simulink model "ctrl_custom_4corner_automatic"  (R2016b)
settings: Solver=ode4  StartTime=0.0  StopTime=inf  FixedStep=0.01  RelTol=1e-3  EnableMultiTasking=on
values from neighbouring files (symbols this model uses):
  alpha = R_T*Eta_t_dot - K1*z_1    [Immersion.m]
undefined symbols (not defined in the file or in its folder): T_pinv_m
libraries: marine_gnc x6, simulink x1
(part 5 of 5)

== system ctrl_custom_4corner_automatic/Complete MPAC1/MPAC Vel/zeta_phi ==
  Constant : Constant  Value=1.2
  Mux : Mux  Inputs=3
  zeta_phi_1 : S-Function  Priority=2  FunctionName=NIVeriStandIO  Parameters=width dtype portnum stime stype btype  SFunctionDeploymentMode=off  EnableBusSupport=off  mask(NI VeriStand Inport){portnum=2, width=-1, stime=-1, dtype=auto, stype=auto, btype=1}
      mask prompts: portnum "Port number:"; width "Port dimensions (-1 for dynamically sized):"; stime "Sample time (-1 for inherited):"; dtype "Data type:"; stype "Signal type:"; btype "Block type:"
      mask help: Use this inport on any level of nested subsystems to allow NI VeriStand software to map signals to it.
      mask init:
      | NIVeriStandIO_init;
      settings: CopyFcn=NIVeriStand_MDL_functions('', 'IO_copy');  DeleteFcn=NIVeriStand_MDL_functions('', 'IO_delete');  MoveFcn=set_param(gcb, 'Mask', 'on');
      mask Callback portnum: NIVeriStand_MDL_functions('', 'IO_setportnum');
      mask TypeOptions dtype: auto | double | single | int8 | uint8 | int16 | uint16 | int32 | uint32 | boolean
      mask Callback dtype: NIVeriStand_MDL_functions('', 'IO_booleansignal');
      mask TypeOptions stype: auto | real | complex
      mask Display:
      | patch([-x x], [-y y], [.90980 .81960 .32156]);
      | plot([xrad -x x xrad], [yrad -y y yrad]);
      | fprintf('NI In%d', portnum);
  zeta_phi_2 : S-Function  Priority=3  FunctionName=NIVeriStandIO  Parameters=width dtype portnum stime stype btype  SFunctionDeploymentMode=off  EnableBusSupport=off  mask(NI VeriStand Inport){portnum=3, width=-1, stime=-1, dtype=auto, stype=auto, btype=1}
      mask prompts: portnum "Port number:"; width "Port dimensions (-1 for dynamically sized):"; stime "Sample time (-1 for inherited):"; dtype "Data type:"; stype "Signal type:"; btype "Block type:"
      mask help: Use this inport on any level of nested subsystems to allow NI VeriStand software to map signals to it.
      mask init:
      | NIVeriStandIO_init;
      settings: CopyFcn=NIVeriStand_MDL_functions('', 'IO_copy');  DeleteFcn=NIVeriStand_MDL_functions('', 'IO_delete');  MoveFcn=set_param(gcb, 'Mask', 'on');
      mask Callback portnum: NIVeriStand_MDL_functions('', 'IO_setportnum');
      mask TypeOptions dtype: auto | double | single | int8 | uint8 | int16 | uint16 | int32 | uint32 | boolean
      mask Callback dtype: NIVeriStand_MDL_functions('', 'IO_booleansignal');
      mask TypeOptions stype: auto | real | complex
      mask Display:
      | patch([-x x], [-y y], [.90980 .81960 .32156]);
      | plot([xrad -x x xrad], [yrad -y y yrad]);
      | fprintf('NI In%d', portnum);
  zeta_phi_3 : S-Function  Priority=1  FunctionName=NIVeriStandIO  Parameters=width dtype portnum stime stype btype  SFunctionDeploymentMode=off  EnableBusSupport=off  mask(NI VeriStand Inport){portnum=1, width=-1, stime=-1, dtype=auto, stype=auto, btype=1}
      mask prompts: portnum "Port number:"; width "Port dimensions (-1 for dynamically sized):"; stime "Sample time (-1 for inherited):"; dtype "Data type:"; stype "Signal type:"; btype "Block type:"
      mask help: Use this inport on any level of nested subsystems to allow NI VeriStand software to map signals to it.
      mask init:
      | NIVeriStandIO_init;
      settings: CopyFcn=NIVeriStand_MDL_functions('', 'IO_copy');  DeleteFcn=NIVeriStand_MDL_functions('', 'IO_delete');  MoveFcn=set_param(gcb, 'Mask', 'on');
      mask Callback portnum: NIVeriStand_MDL_functions('', 'IO_setportnum');
      mask TypeOptions dtype: auto | double | single | int8 | uint8 | int16 | uint16 | int32 | uint32 | boolean
      mask Callback dtype: NIVeriStand_MDL_functions('', 'IO_booleansignal');
      mask TypeOptions stype: auto | real | complex
      mask Display:
      | patch([-x x], [-y y], [.90980 .81960 .32156]);
      | plot([xrad -x x xrad], [yrad -y y yrad]);
      | fprintf('NI In%d', portnum);
  zeta_phi : Outport
  wires:
  zeta_phi_1/1 -> Mux/1
  zeta_phi_3/1 -> Mux/3
  zeta_phi_2/1 -> Mux/2
  Constant/1 -> zeta_phi/1

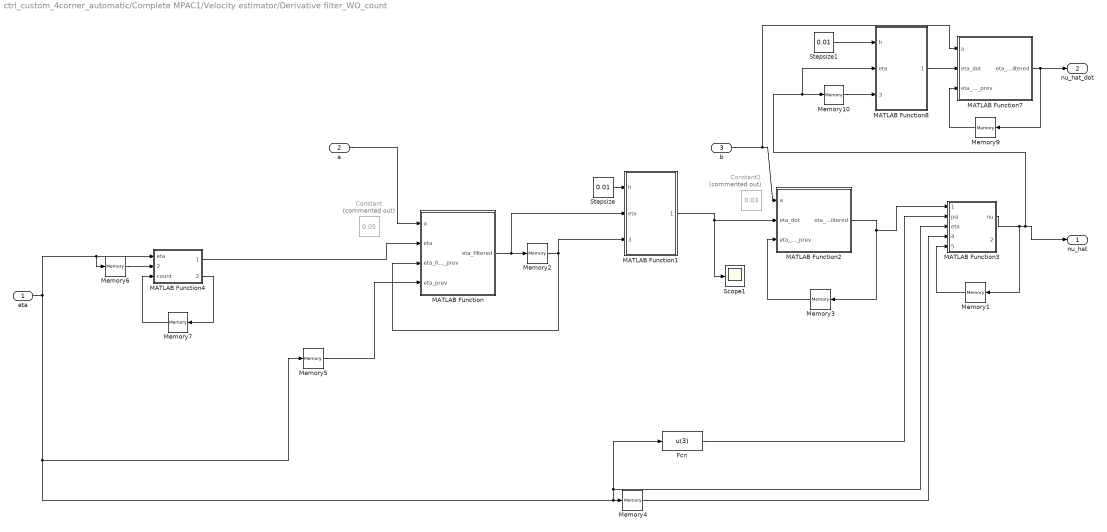
== system ctrl_custom_4corner_automatic/Complete MPAC1/Velocity estimator/Derivative filter_WO_count ==
  eta : Inport
  a : Inport  Port=2
  b : Inport  Port=3
  Constant : Constant  Commented=on  Value=0.05
  Constant2 : Constant  Commented=on  Value=0.03
  Fcn : Fcn  Expr=u(3)
  MATLAB Function : MATLAB Function  TreatAsAtomicUnit=on
  MATLAB Function1 : MATLAB Function  TreatAsAtomicUnit=on
  MATLAB Function2 : MATLAB Function  TreatAsAtomicUnit=on
  MATLAB Function3 : MATLAB Function  TreatAsAtomicUnit=on
  MATLAB Function4 : MATLAB Function  TreatAsAtomicUnit=on
  MATLAB Function7 : MATLAB Function  TreatAsAtomicUnit=on
  MATLAB Function8 : MATLAB Function  TreatAsAtomicUnit=on
  Memory{1..6,9..10} (8 alike) : Memory  X0=[0 0 0]
  Memory7 : Memory
  Scope1 : Scope
  Stepsize : Constant  Value=0.01
  Stepsize1 : Constant  Value=0.01
  nu_hat : Outport
  nu_hat_dot : Outport  Port=2
  wires:
  MATLAB Function7/1(eta_dot_filtered) -> Memory9/1, nu_hat_dot/1
  MATLAB Function4/2(count_out) -> Memory7/1
  Memory7/1 -> MATLAB Function4/3(count)
  Memory6/1 -> MATLAB Function4/2(eta_prev)
  MATLAB Function4/1(eta_out) -> MATLAB Function/2(eta)
  Stepsize1/1 -> MATLAB Function8/1(h)
  Memory10/1 -> MATLAB Function8/3(eta_prev)
  MATLAB Function8/1(eta_dot) -> MATLAB Function7/2(eta_dot)
  Memory9/1 -> MATLAB Function7/3(eta_dot_filtered_prev)
  eta/1 -> MATLAB Function4/1(eta), Memory6/1, Memory4/1, MATLAB Function3/3(eta), Fcn/1, Memory5/1
  Memory5/1 -> MATLAB Function/4(eta_prev)
  MATLAB Function3/1(nu) -> nu_hat/1, Memory10/1, MATLAB Function8/2(eta), Memory1/1
  Memory4/1 -> MATLAB Function3/4(prev_eta)
  Memory1/1 -> MATLAB Function3/5(prev_nu)
  MATLAB Function/1(eta_filtered) -> Memory2/1, MATLAB Function1/2(eta)
  b/1 -> MATLAB Function2/1(a), MATLAB Function7/1(a)
  a/1 -> MATLAB Function/1(a)
  Memory3/1 -> MATLAB Function2/3(eta_dot_filtered_prev)
  MATLAB Function2/1(eta_dot_filtered) -> Memory3/1, MATLAB Function3/1(eta_dot)
  MATLAB Function1/1(eta_dot) -> MATLAB Function2/2(eta_dot), Scope1/1
  Memory2/1 -> MATLAB Function/3(eta_filtered_prev), MATLAB Function1/3(eta_prev)
  Stepsize/1 -> MATLAB Function1/1(h)
  Fcn/1 -> MATLAB Function3/2(psi)

== system ctrl_custom_4corner_automatic/Saturation/MRS_num/LP ==
  In1 : Inport
  Gain1 : Gain  Gain=2  Multiplication=Matrix(K*u)
  Integrator : Integrator  InitialCondition=[0;0;0]
  Sum2 : Sum  Inputs=|+-
  Out1 : Outport
  wires:
  Sum2/1 -> Gain1/1
  In1/1 -> Sum2/1
  Integrator/1 -> Sum2/2, Out1/1
  Gain1/1 -> Integrator/1

== system ctrl_custom_4corner_automatic/Saturation1/MRS_num/LP ==
  In1 : Inport
  Gain1 : Gain  Gain=2  Multiplication=Matrix(K*u)
  Integrator : Integrator  InitialCondition=[0;0;0]
  Sum2 : Sum  Inputs=|+-
  Out1 : Outport
  wires:
  Gain1/1 -> Integrator/1
  Integrator/1 -> Out1/1, Sum2/2
  In1/1 -> Sum2/1
  Sum2/1 -> Gain1/1

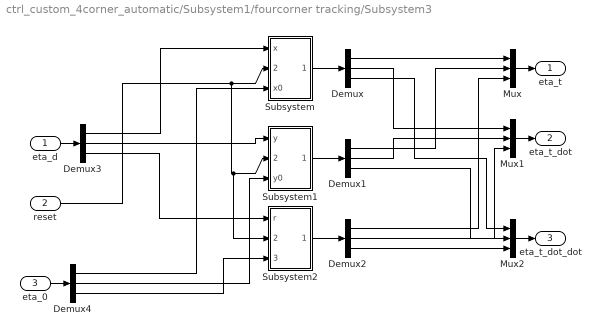
== system ctrl_custom_4corner_automatic/Subsystem1/fourcorner tracking/Subsystem3 ==
  eta_d : Inport
  reset : Inport  Port=2
  eta_0 : Inport  Port=3
  Demux{,1..4} (5 alike) : Demux  Outputs=3
  Mux : Mux  Inputs=3
  Mux1 : Mux  Inputs=3
  Mux2 : Mux  Inputs=3
  Subsystem : Subsystem
  Subsystem1 : Subsystem
  Subsystem2 : Subsystem
  eta_t : Outport  PortDimensions=3
  eta_t_dot : Outport  Port=2  PortDimensions=3
  eta_t_dot_dot : Outport  Port=3  PortDimensions=3
  wires:
  Subsystem1/1(y,yd,ydd) -> Demux1/1
  Subsystem2/1(y,yd,ydd) -> Demux2/1
  Subsystem/1(x,xd,xdd) -> Demux/1
  Demux/3 -> Mux2/1
  eta_d/1 -> Demux3/1
  Mux1/1 -> eta_t_dot/1
  Demux/1 -> Mux/1
  Mux2/1 -> eta_t_dot_dot/1
  Demux3/1 -> Subsystem/1(x)
  Demux1/3 -> Mux2/2
  Demux2/3 -> Mux2/3
  Demux1/1 -> Mux/2
  Demux3/2 -> Subsystem1/1(y)
  Demux3/3 -> Subsystem2/1(r)
  Demux2/2 -> Mux1/3
  Demux1/2 -> Mux1/2
  reset/1 -> Subsystem2/2(reset), Subsystem1/2(reset), Subsystem/2(reset)
  Mux/1 -> eta_t/1
  Demux/2 -> Mux1/1
  Demux2/1 -> Mux/3
  Demux4/3 -> Subsystem2/3(psi0)
  Demux4/2 -> Subsystem1/3(y0)
  Demux4/1 -> Subsystem/3(x0)
  eta_0/1 -> Demux4/1

== system ctrl_custom_4corner_automatic/Complete MPAC1/MPAC/Subsystem/10HZ ==
  In1 : Inport
  MATLAB Function : MATLAB Function  TreatAsAtomicUnit=on
  Memory : Memory
  Memory1 : Memory
  Out1 : Outport
  wires:
  Memory/1 -> MATLAB Function/3(i)
  MATLAB Function/2(i_out) -> Memory/1
  Memory1/1 -> MATLAB Function/2(nu_current)
  MATLAB Function/1(nu_10) -> Out1/1, Memory1/1
  In1/1 -> MATLAB Function/1(nu)

== system ctrl_custom_4corner_automatic/Subsystem1/fourcorner tracking/Subsystem3/Subsystem ==
  x : Inport
  reset : Inport  Port=2
  x0 : Inport  Port=3
  Constant : Constant  Value=0
  Gain1 : Gain  Gain=[0 0 0.0017]'  Multiplication=Matrix(K*u)
  Gain2 : Gain  Gain=[1 0 0;0 1 0;0 0 1]  Multiplication=Matrix(K*u)
  Gain3 : Gain  Gain=[0 1 0;0 0 1;-0.0017 -0.049 -0.408]  Multiplication=Matrix(K*u)
  Integrator : Integrator  ExternalReset=either  InitialConditionSource=external
  Mux : Mux  Inputs=3
  Sum : Sum  Inputs=|++
  x,xd,xdd : Outport  PortDimensions=3
  wires:
  Gain1/1 -> Sum/1
  x/1 -> Gain1/1
  Integrator/1 -> Gain2/1, Gain3/1
  Sum/1 -> Integrator/1
  Gain2/1 -> x,xd,xdd/1
  Mux/1 -> Integrator/3
  reset/1 -> Integrator/2
  Gain3/1 -> Sum/2
  Constant/1 -> Mux/2, Mux/3
  x0/1 -> Mux/1

== system ctrl_custom_4corner_automatic/Subsystem1/fourcorner tracking/Subsystem3/Subsystem1 ==
  y : Inport
  reset : Inport  Port=2
  y0 : Inport  Port=3
  Constant : Constant  Value=0
  Gain1 : Gain  Gain=[0 0 0.0017]'  Multiplication=Matrix(K*u)
  Gain2 : Gain  Gain=[1 0 0;0 1 0;0 0 1]  Multiplication=Matrix(K*u)
  Gain3 : Gain  Gain=[0 1 0;0 0 1;-0.0017 -0.049 -0.408]  Multiplication=Matrix(K*u)
  Integrator : Integrator  ExternalReset=either  InitialConditionSource=external
  Mux : Mux  Inputs=3
  Sum : Sum  Inputs=|++
  y,yd,ydd : Outport
  wires:
  Constant/1 -> Mux/3, Mux/2
  Gain3/1 -> Sum/2
  reset/1 -> Integrator/2
  Mux/1 -> Integrator/3
  Gain2/1 -> y,yd,ydd/1
  Sum/1 -> Integrator/1
  Integrator/1 -> Gain3/1, Gain2/1
  y/1 -> Gain1/1
  Gain1/1 -> Sum/1
  y0/1 -> Mux/1

== system ctrl_custom_4corner_automatic/Subsystem1/fourcorner tracking/Subsystem3/Subsystem2 ==
  r : Inport
  reset : Inport  Port=2
  psi0 : Inport  Port=3
  Constant : Constant  Value=0
  Gain1 : Gain  Gain=[0 0 0.0017]'  Multiplication=Matrix(K*u)
  Gain2 : Gain  Gain=[1 0 0;0 1 0;0 0 1]  Multiplication=Matrix(K*u)
  Gain3 : Gain  Gain=[0 1 0;0 0 1;-0.0017 -0.049 -0.408]  Multiplication=Matrix(K*u)
  Integrator : Integrator  ExternalReset=either  InitialConditionSource=external
  Mux : Mux  Inputs=3
  Sum : Sum  Inputs=|++
  y,yd,ydd : Outport
  wires:
  Gain1/1 -> Sum/1
  r/1 -> Gain1/1
  Integrator/1 -> Gain2/1, Gain3/1
  Sum/1 -> Integrator/1
  Gain2/1 -> y,yd,ydd/1
  Mux/1 -> Integrator/3
  reset/1 -> Integrator/2
  Gain3/1 -> Sum/2
  Constant/1 -> Mux/2, Mux/3
  psi0/1 -> Mux/1

== matlab function ctrl_custom_4corner_automatic/Projection [-pi,pi] to [-inf,inf] + shortest rotation/MATLAB Function11 ==
  data: alpha_prev input; alpha_infinf output; alpha_pipi input
function alpha_infinf  = fcn(alpha_prev,alpha_pipi)
alpha_infinf = NaN(6,1);

for i = 1:6
    % current rotation
    n = sign(alpha_prev(i)) * fix( (abs(alpha_prev(i))+pi)/(2*pi) ); 

    alpha_infinf(i) = 2*pi*n + alpha_pipi(i);

    alpha_tilde = alpha_infinf(i) - alpha_prev(i);

    % Shortest rotation
    if abs(alpha_tilde)>pi
        alpha_infinf(i) = alpha_infinf(i) - sign(alpha_tilde)*2*pi;
    end
end

end

== matlab function ctrl_custom_4corner_automatic/Input1/Control Gains/MATLAB Function ==
  data: u input; y output
function y = fcn(u)

y = diag(u);

== matlab function ctrl_custom_4corner_automatic/Thrust allocation: Pseudo-inverse of extended thrust configuration matrix/MATLAB Function11 ==
  data: u_e input; u output
function u   = fcn(u_e)
u = [norm(u_e( 1: 2))
     norm(u_e( 3: 4))
     norm(u_e( 5: 6))
     norm(u_e( 7: 8))
     norm(u_e( 9:10))
     norm(u_e(11:12))];

%{
alpha = [atan2(u_e( 2),u_e( 1))
         atan2(u_e( 4),u_e( 3))
         atan2(u_e( 6),u_e( 5))
         atan2(u_e( 8),u_e( 7))
         atan2(u_e(10),u_e( 9))
         atan2(u_e(12),u_e(11))];
%}
end

== matlab function ctrl_custom_4corner_automatic/Input1/Control Gains/MATLAB Function1 ==
  data: u input; y output
function y = fcn(u)

y = diag(u);

== matlab function ctrl_custom_4corner_automatic/Input1/Control Gains/MATLAB Function2 ==
  data: u input; y output
function y = fcn(u)

y = diag(u);

== matlab function ctrl_custom_4corner_automatic/diag ==
  data: w_d output; w_d1 input
function w_d = fcn(w_d1)
%#codegen

w_d = diag([w_d1,w_d1,w_d1]);

== matlab function ctrl_custom_4corner_automatic/diag1 ==
  data: w_d output; w_d1 input
function w_d = fcn(w_d1)
%#codegen

w_d = diag([w_d1,w_d1,w_d1]);

== matlab function ctrl_custom_4corner_automatic/Complete MPAC1/10HZ/MATLAB Function ==
  data: nu input; nu_10 output; nu_current input; i input; i_out output
function [nu_10,i_out] = hz(nu,nu_current,i)

if i==0
    nu_10=nu;
    i_out=1;
elseif i==10
    nu_10=nu;
    i_out=1;
else
    nu_10=nu_current;
    i_out=i+1;
end

== matlab function ctrl_custom_4corner_automatic/Complete MPAC1/MPAC/MATLAB Function ==
  data: theta_dot output; L1 input; nu_p_dot output; L2 input; nu input; tau input; theta input; nu_p input
function [theta_dot,nu_p_dot] = MPAC(L1,L2,nu,tau,theta,nu_p)

m = 127.92;%14.79;
x_g = 0;%0.0375;
I_z = 61.967;%1.7600;  

X_ud = -3.262; %-2.0;                                           % Table B.1
Y_vd = -28.89;%-10.0;
N_vd = -0.157;%-0.0;     % Table B.1
Y_rd = -0.525;%  -0.0;
N_rd = -13.98;%-1.0;     % Table B.1

M_RB_c=[m 0 0;...
0 m m*x_g;...
0 m*x_g I_z];
M_A_c=[-X_ud 0 0;...
0 -Y_vd -Y_rd;...
0 -N_vd -N_rd];
M=M_RB_c+M_A_c;

X_u = -2.33;
Y_v = -4.67;
Y_r = -7.25;
N_v = 0;
N_r = -0.0168;

D = [-X_u 0 0; 0 -Y_v -Y_r; 0 -N_v -N_r];



nu_tilde = nu_p-nu;
nu_p_dot = M^(-1)*(tau+theta-D*nu_p-L1*nu_tilde);
theta_dot = -L2*nu_tilde;

== matlab function ctrl_custom_4corner_automatic/Complete MPAC1/MPAC/MATLAB Function1 ==
  data: L1 output; omega_theta input; L2 output; zeta_theta input
function [L1, L2] = MPAC_GAIN(omega_theta,zeta_theta)

m = 127.92;%14.79;
x_g = 0;%0.0375;
I_z = 61.967;%1.7600;  

X_ud = -3.262; %-2.0;                                           % Table B.1
Y_vd = -28.89;%-10.0;
N_vd = -0.157;%-0.0;     % Table B.1
Y_rd = -0.525;%  -0.0;
N_rd = -13.98;%-1.0;     % Table B.1

M_RB_c=[m 0 0;...
0 m m*x_g;...
0 m*x_g I_z];
M_A_c=[-X_ud 0 0;...
0 -Y_vd -Y_rd;...
0 -N_vd -N_rd];
M=M_RB_c+M_A_c;

M_diag=diag(M);

L1 = 2*diag(zeta_theta)*diag(omega_theta)*diag(M_diag);
L2 = diag(omega_theta)^2*diag(M_diag);

== matlab function ctrl_custom_4corner_automatic/Complete MPAC1/MPAC Vel/MATLAB Function3 ==
  data: kappa1 output; omega_phi input; kappa2 output; zeta_phi input
function [kappa1, kappa2] = MPAC_GAIN_Vel(omega_phi,zeta_phi)

kappa1 = 2*diag(zeta_phi)*diag(omega_phi)*eye(3);
kappa2 = diag(omega_phi)^2*eye(3);

== matlab function ctrl_custom_4corner_automatic/Complete MPAC1/MPAC Vel/MATLAB Function2 ==
  data: Phi_p_dot output; kappa1 input; eta_p_dot output; kappa2 input; eta input; Phi_p input; eta_p input
function [Phi_p_dot,eta_p_dot] = MPAC_Vel(kappa1,kappa2,eta,Phi_p,eta_p)

eta_tilde = eta_p-eta;
eta_p_dot = Phi_p-kappa1*eta_tilde;
Phi_p_dot = -kappa2*eta_tilde;

== matlab function ctrl_custom_4corner_automatic/Control/Gamma_theta/MATLAB Function1 ==
  data: K_p output; K_p1 input
function K_p = fcn(K_p1)
%#codegen

K_p = diag(K_p1);

== matlab function ctrl_custom_4corner_automatic/Complete MPAC1/Velocity estimator/Derivative filter_WO_count/MATLAB Function ==
  data: a input; eta_filtered output; eta input; eta_filtered_prev input; eta_prev input
function eta_filtered  = fcn(a,eta,eta_filtered_prev,eta_prev)

psi = eta(3);
psitilde = psi-eta_prev(3);


eta_filtered = a*eta + (1-a)*eta_filtered_prev;

== matlab function ctrl_custom_4corner_automatic/Complete MPAC1/Velocity estimator/Derivative filter_WO_count/MATLAB Function1 ==
  data: h input; eta_dot output; eta input; eta_prev input
function eta_dot  = fcn(h,eta,eta_prev)

eta_tilde = eta-eta_prev;
eta_dot = (eta_tilde)./h;

if eta_dot(3)>5;
    eta_dot(3)=5;
elseif eta_dot(3)<-5;
   eta_dot(3)=-5; 
end

== matlab function ctrl_custom_4corner_automatic/Input1/Guidance gains/MATLAB Function ==
  data: u input; y output
function y = fcn(u)

y = diag(u);

== matlab function ctrl_custom_4corner_automatic/Input1/Guidance gains/MATLAB Function1 ==
  data: u input; y output
function y = fcn(u)

y = diag(u);

== matlab function ctrl_custom_4corner_automatic/Complete MPAC1/Velocity estimator/Derivative filter_WO_count/MATLAB Function2 ==
  data: a input; eta_dot_filtered output; eta_dot input; eta_dot_filtered_prev input
function eta_dot_filtered = fcn(a,eta_dot,eta_dot_filtered_prev)

eta_dot_filtered = a*eta_dot + (1-a)*eta_dot_filtered_prev;

== matlab function ctrl_custom_4corner_automatic/Complete MPAC1/Velocity estimator/Derivative filter_WO_count/MATLAB Function3 ==
  data: eta_dot input; nu output; psi input; eta input; prev_eta input; prev_nu input; count_out output
function [nu,count_out] = fcn(eta_dot,psi,eta,prev_eta,prev_nu)


if(prev_eta(1)==eta(1)||prev_eta(2)==eta(2)||prev_eta(3)==eta(3))
    nu = prev_nu;
    count_out =1;
else
    %if count == 1
        %nu = prev_nu;
        %count_out = 0;
    %else
        R_inv = [cos(psi)  sin(psi) 0
                 -sin(psi) cos(psi) 0
                 0         0        1];
        nu = R_inv*eta_dot;
        count_out = 0;
    %end
end

== matlab function ctrl_custom_4corner_automatic/Complete MPAC1/Velocity estimator/Derivative filter_WO_count/MATLAB Function4 ==
  data: eta input; eta_out output; eta_prev input; count input; count_out output
function [eta_out,count_out] = fcn(eta,eta_prev,count)

angle_d = eta(3)*180/pi;%+count*360;
angle = eta_prev(3)*180/pi;%+count*360;

angle_tilde = angle_d-angle;

if abs(angle_tilde)>300;
    count_out=-sign(angle_tilde)+count;
    angle_out=angle_d+count_out*360;
else
    count_out=count;
    angle_out=angle_d+count_out*360;
end

eta_out = eta;
eta_out(3) = angle_out*pi/180;


end

== matlab function ctrl_custom_4corner_automatic/Complete MPAC1/Velocity estimator/Derivative filter_WO_count/MATLAB Function7 ==
  data: a input; eta_dot_filtered output; eta_dot input; eta_dot_filtered_prev input
function eta_dot_filtered = fcn(a,eta_dot,eta_dot_filtered_prev)

eta_dot_filtered = a*eta_dot + (1-a)*eta_dot_filtered_prev;

== matlab function ctrl_custom_4corner_automatic/Complete MPAC1/Velocity estimator/Derivative filter_WO_count/MATLAB Function8 ==
  data: h input; eta_dot output; eta input; eta_prev input
function eta_dot  = fcn(h,eta,eta_prev)

eta_tilde = eta-eta_prev;
eta_dot = (eta_tilde)./h;

if eta_dot(3)>5;
    eta_dot(3)=5;
elseif eta_dot(3)<-5;
   eta_dot(3)=-5; 
end

== matlab function ctrl_custom_4corner_automatic/Guidance1/Reference model/w_d*w_d ==
  data: w_d input; y output
function y = fcn(w_d)
%#codegen

y = w_d*w_d;

== matlab function ctrl_custom_4corner_automatic/Input1/Observer Gains/MATLAB Function ==
  data: u input; y output
function y = fcn(u)

y = diag(u);

== matlab function ctrl_custom_4corner_automatic/Complete MPAC1/Velocity estimator/wraphandle ==
  data: eta input; eta_out output; eta_prev input; count input; count_out output
function [eta_out,count_out] = fcn(eta,eta_prev,count)

angle_d = eta(3)*180/pi;%+count*360;
angle = eta_prev(3)*180/pi;%+count*360;

angle_tilde = angle_d-angle;

if abs(angle_tilde)>300;
    count_out=-sign(angle_tilde)+count;
    angle_out=angle_d+count_out*360;
else
    count_out=count;
    angle_out=angle_d+count_out*360;
end

eta_out = eta;
eta_out(3) = angle_out*pi/180;


end

== matlab function ctrl_custom_4corner_automatic/Guidance1/Reference model/w_d*w_d1 ==
  data: w_d input; y output; zeta input
function y = fcn(w_d,zeta)
%#codegen

y = 2*zeta*w_d;

== matlab function ctrl_custom_4corner_automatic/Guidance1/Reference model/w_d^-2 ==
  data: w_d input; y output
function y = fcn(w_d)
%#codegen

y = w_d^-2;

== matlab function ctrl_custom_4corner_automatic/Guidance1/Reference model/w_d^3 ==
  data: w_d input; y output
function y = fcn(w_d)
%#codegen

y = w_d^3;

== matlab function ctrl_custom_4corner_automatic/10HZ/MATLAB Function ==
  data: nu input; nu_10 output; nu_current input; i input; i_out output
function [nu_10,i_out] = hz(nu,nu_current,i)

if i==0
    nu_10=nu;
    i_out=1;
elseif i==10
    nu_10=nu;
    i_out=1;
else
    nu_10=nu_current;
    i_out=i+1;
end

== matlab function ctrl_custom_4corner_automatic/Input1/Observer Gains/MATLAB Function1 ==
  data: u input; y output
function y = fcn(u)

y = diag(u);

== matlab function ctrl_custom_4corner_automatic/Input1/Observer Gains/MATLAB Function2 ==
  data: u input; y output
function y = fcn(u)

y = diag(u);

== matlab function ctrl_custom_4corner_automatic/10HZ1/MATLAB Function ==
  data: nu input; nu_10 output; nu_current input; i input; i_out output
function [nu_10,i_out] = hz(nu,nu_current,i)

if i==0
    nu_10=nu;
    i_out=1;
elseif i==10
    nu_10=nu;
    i_out=1;
else
    nu_10=nu_current;
    i_out=i+1;
end

== matlab function ctrl_custom_4corner_automatic/Control/K1/MATLAB Function ==
  data: K_p output; K_p1 input
function K_p = fcn(K_p1)
%#codegen

K_p = diag(K_p1);

== matlab function ctrl_custom_4corner_automatic/10HZ2/MATLAB Function ==
  data: nu input; nu_10 output; nu_current input; i input; i_out output
function [nu_10,i_out] = hz(nu,nu_current,i)

if i==0
    nu_10=nu;
    i_out=1;
elseif i==10
    nu_10=nu;
    i_out=1;
else
    nu_10=nu_current;
    i_out=i+1;
end

== matlab function ctrl_custom_4corner_automatic/10HZ3/MATLAB Function ==
  data: nu input; nu_10 output; nu_current input; i input; i_out output
function [nu_10,i_out] = hz(nu,nu_current,i)

if i==0
    nu_10=nu;
    i_out=1;
elseif i==10
    nu_10=nu;
    i_out=1;
else
    nu_10=nu_current;
    i_out=i+1;
end

== matlab function ctrl_custom_4corner_automatic/10HZ4/MATLAB Function ==
  data: nu input; nu_10 output; nu_current input; i input; i_out output
function [nu_10,i_out] = hz(nu,nu_current,i)

if i==0
    nu_10=nu;
    i_out=1;
elseif i==10
    nu_10=nu;
    i_out=1;
else
    nu_10=nu_current;
    i_out=i+1;
end

== matlab function ctrl_custom_4corner_automatic/Control/10HZ/MATLAB Function ==
  data: nu input; nu_10 output; nu_current input; i input; i_out output
function [nu_10,i_out] = hz(nu,nu_current,i)

if i==0
    nu_10=nu;
    i_out=1;
elseif i==10
    nu_10=nu;
    i_out=1;
else
    nu_10=nu_current;
    i_out=i+1;
end

== matlab function ctrl_custom_4corner_automatic/Control/K2/MATLAB Function1 ==
  data: K_p output; K_p1 input
function K_p = fcn(K_p1)
%#codegen

K_p = diag(K_p1);

== matlab function ctrl_custom_4corner_automatic/10HZ5/MATLAB Function ==
  data: nu input; nu_10 output; nu_current input; i input; i_out output
function [nu_10,i_out] = hz(nu,nu_current,i)

if i==0
    nu_10=nu;
    i_out=1;
elseif i==10
    nu_10=nu;
    i_out=1;
else
    nu_10=nu_current;
    i_out=i+1;
end

== matlab function ctrl_custom_4corner_automatic/Complete MPAC1/MPAC/Subsystem/MATLAB Function ==
  data: gain input; u input; y output
function y = fcn(gain,u)

y = u/gain;

== matlab function ctrl_custom_4corner_automatic/10HZ6/MATLAB Function ==
  data: nu input; nu_10 output; nu_current input; i input; i_out output
function [nu_10,i_out] = hz(nu,nu_current,i)

if i==0
    nu_10=nu;
    i_out=1;
elseif i==10
    nu_10=nu;
    i_out=1;
else
    nu_10=nu_current;
    i_out=i+1;
end

== matlab function ctrl_custom_4corner_automatic/10HZ7/MATLAB Function ==
  data: nu input; nu_10 output; nu_current input; i input; i_out output
function [nu_10,i_out] = hz(nu,nu_current,i)

if i==0
    nu_10=nu;
    i_out=1;
elseif i==10
    nu_10=nu;
    i_out=1;
else
    nu_10=nu_current;
    i_out=i+1;
end

== matlab function ctrl_custom_4corner_automatic/Control/MATLAB Function4 ==
  data: tau input; dwc_enable output; Eta input; tau1 output; z_1 output; tau_L output; tau_U output; Chi_tilde output; nu input; Eta_t input; Eta_tdot input; Eta_tdotdot input; z_2 output; K_p input; K_d input; Gamma_theta input; delta input; theta_hat input; control_select input; adaptation input; theta_hat_dot output; tau_nom output; Alpha_1 output; w_delta_hat_dot output; eta_hat_dot output; nu_hat_dot output; w_delta_hat input; eta_hat input; nu_hat input; phi_hat input; phi_dot_hat output
   function [dwc_enable, tau1,z_1,tau_L,tau_U,Chi_tilde,z_2,theta_hat_dot,tau_nom,Alpha_1,w_delta_hat_dot,eta_hat_dot,nu_hat_dot,phi_dot_hat] = Cascaded_feedback_controller(tau,Eta,nu,Eta_t,Eta_tdot,Eta_tdotdot,K_p,K_d,Gamma_theta,delta,theta_hat,control_select,adaptation,w_delta_hat,eta_hat,nu_hat,phi_hat)
%  [ tau,theta ] = Adaptiv_controller(Eta,nu,nu_dot,phi,theta_t,Eta_d,Eta_dtheta,Eta_dtheta2,v_s,v_stheta,v_st,h)
%UNTITLED6 Summary of this function goes here Skjetne
%   Detailed explanation goes here
%kan være den må løses på en smartere måte
%include Model_c to path
%#codegen
persistent PHI OMEGA_N EPSI_RR EPSI_PHI RR PHIPHI p_r p_p S_old_RR S_old_PHI pp YY_r YY_phi 


stored_data=20;
if (isempty(PHI)||isempty(OMEGA_N))
    PHI=zeros(8,1);
    OMEGA_N=zeros(3,1);
    PHIPHI=zeros(8,3*stored_data);
    RR=zeros(3,3*stored_data);
    EPSI_RR=zeros(3*stored_data,1);
    EPSI_PHI=zeros(3*stored_data,1);
    S_old_RR=0;
    S_old_PHI=0;
    p_r=1;
    p_p=1;
    pp=1;
    YY_r=zeros(3*stored_data,1);
    YY_phi=zeros(3*stored_data,1);
    
end
Nu_d_DWC = [0 0 0];
dwc_enable = 0;
w_delta_hat_dot= [0 0 0]';
eta_hat_dot= [0 0 0]';
nu_hat_dot= [0 0 0]';
z_1=[0 0 0]';
z_2=[0 0 0]';
%%Model
 X_u		= -2.332;		
X_uu 	=  0;		
X_uuu	= -8.557;

Y_v		= -4.673;   
Y_vv	= -0.3976;
Y_vvv	= -313.3;	
Y_r		= -7.25;
Y_rr	= -3.45;
Y_rrr   = 0;

N_v		= 0;		
N_vv	= -0.2088;
N_vvv = 0;

N_r		= -6.9161;
N_rr	= -4.7342;
N_rrr	= -0.1474;

N_rv	= 0.08;	
N_vr	= 0.08;
Y_rv	= -0.805;			
Y_vr	= -0.845;

X_ud =     -3.262;
Y_vd =     -28.89;
Y_rd =     -0.525;
N_vd =     -0.157;	
N_rd =     -13.98;

Nur  = -Y_rd;
Nuv  = -(Y_vd-X_ud);
Yur  = -X_ud;

x_g     = 0.0375;
m       = 127.92;
I_z     = 61.967;

u   = nu(1);
v   = nu(2);
r   = nu(3);

d_11 = - X_u - X_uu*abs(u) - X_uuu*u^2;
d_22 = - Y_v - Y_vv*abs(v) - Y_rv*abs(r) - Y_vvv*v^2;
d_23 = - Y_r - Y_rr*abs(r) - Y_vr*abs(v) - Y_rrr*r^2 - Yur*u;
d_32 = - N_v - N_vv*abs(v) - N_rv*abs(r) - N_vvv*v^2 - Nuv*u;
d_33 = - N_r - N_rr*abs(r) - N_vr*abs(v) - N_rrr*r^2 - Nur*u;

D    = [d_11  0     0
        0     d_22  d_23
        0     d_32  d_33];

CA=[0                            0          Y_vd*v+Y_rd*r;
    0                            0                -X_ud*u;
    -Y_rd*r-Y_vd*v               X_ud*u                0];

CRB=[0             0     -m*(x_g*r+v);
     0             0      m*u;
     m*(x_g*r+v) -m*u     0]; 

C=CRB+CA;

M_RB_c=[m     0      0;
        0     m      m*x_g;
        0     m*x_g  I_z];

M_A_c=[-X_ud    0      0;
         0    -Y_vd  -Y_rd;
         0    -N_vd  -N_rd];     
    
M_c = M_RB_c + M_A_c;

%model end 
psi = Eta(3);
r = nu(3);

S = [0 -r  0; r  0  0; 0  0  0];
S_T = S';
R = [cos(psi) -sin(psi) 0; sin(psi) cos(psi) 0; 0 0 1];
R_T = R';
    
%% controlsignaler
Eta_tilde=Eta-Eta_t;
Chi_tilde=Eta(3)-Eta_t(3);
Chi_tilde=mod(pi/2+Chi_tilde,pi)-pi/2; %%%%%%%%%%%%%%%%%%%%%%

%% New Controller

switch control_select
    case 1 %DWC - NPLV
        %NPLV-tanh
        z_1=R'*(Eta_tilde);
        Delta_1 = diag([delta(1) delta(1) delta(2)]);

        Alpha_1=(-K_p*tanh(Delta_1^(-1)*z_1)+(R')*Eta_tdot);
        z_2=nu-Alpha_1;

        z_1_dot=S(nu)'*z_1-K_p*tanh(Delta_1^(-1)*z_1)+z_2;
        
        
        Alpha_1dot=-K_p*(ones(3,1)-(tanh(Delta_1^(-1)*z_1)).^2).*(Delta_1^(-1)*z_1_dot)+S(nu)'*R'*Eta_tdot + R'*Eta_tdotdot;

        % TAU 
        %tau=M_c*Alpha_1dot-K_d*z_2;
        %theta_hat_dot = [0 0 0]';
        
        switch adaptation
            case 1
                tau=M_c*Alpha_1dot-K_d*z_2-theta_hat;
                theta_hat_dot = Gamma_theta*z_2;
                tau_nom =M_c*Alpha_1dot-K_d*z_2;
            otherwise
                tau=M_c*Alpha_1dot-K_d*z_2;
                theta_hat_dot = [0 0 0]';
                tau_nom =M_c*Alpha_1dot-K_d*z_2;
        end 
        
        
    case 2
        %NPLV
        z_1=R'*(Eta_tilde);

        E1 = eye(2)/sqrt([z_1(1) z_1(2)]*[z_1(1) z_1(2)]'+delta(1)^2);
        E2 = 1/sqrt(z_1(3)^2+delta(2)^2);

        K_1z1Delta = K_p*([E1 zeros(2,1); zeros(1,2) E2]);

        Alpha_1=(-K_1z1Delta*z_1+(R')*Eta_tdot);
        z_2=nu-Alpha_1;

        z_1_dot=S(nu)'*z_1-K_1z1Delta*z_1+z_2;
        dz_1 = z_1_dot;
        E3 = [z_1(1) z_1(2)]*[dz_1(1) dz_1(2)]'/([z_1(1) z_1(2)]*[z_1(1) z_1(2)]'+delta(1)^2)^(3/2)*eye(2);
        E4 = z_1(3)*dz_1(3)/sqrt(z_1(3)^2+delta(2)^2);

        Dot_K_1z1Delta = -K_p*([E3 zeros(2,1); zeros(1,2) E4]);


        Alpha_1dot=-(Dot_K_1z1Delta*z_1+K_1z1Delta*z_1_dot)+S(nu)'*R'*Eta_tdot + R'*Eta_tdotdot;

        % TAU 
        %tau=M_c*Alpha_1dot-K_d*z_2;
        %theta_hat_dot = [0 0 0]';
        
        switch adaptation
            case 1
                tau=M_c*Alpha_1dot-K_d*z_2-theta_hat;
                theta_hat_dot = Gamma_theta*z_2;
                tau_nom =M_c*Alpha_1dot-K_d*z_2;
            otherwise
                tau=M_c*Alpha_1dot +C*Alpha_1 + D*Alpha_1 - K_d*z_2;
                theta_hat_dot = [0 0 0]';
                tau_nom =M_c*Alpha_1dot-K_d*z_2;
        end
    case 3
        %NPNV
        z_1=R'*(Eta_tilde);

        E1 = eye(2)/sqrt([z_1(1) z_1(2)]*[z_1(1) z_1(2)]'+delta(1)^2);
        E2 = 1/sqrt(z_1(3)^2+delta(2)^2);

        K_1z1Delta = K_p*([E1 zeros(2,1); zeros(1,2) E2]);

        Alpha_1=(-K_1z1Delta*z_1+(R')*Eta_tdot);
        z_2=nu-Alpha_1;

        z_1_dot=S(nu)'*z_1-K_1z1Delta*z_1+z_2;
        dz_1 = z_1_dot;
        E3 = [z_1(1) z_1(2)]*[dz_1(1) dz_1(2)]'/([z_1(1) z_1(2)]*[z_1(1) z_1(2)]'+delta(1)^2)^(3/2)*eye(2);
        E4 = z_1(3)*dz_1(3)/sqrt(z_1(3)^2+delta(2)^2);

        Dot_K_1z1Delta = -K_p*([E3 zeros(2,1); zeros(1,2) E4]);


        Alpha_1dot=-(Dot_K_1z1Delta*z_1+K_1z1Delta*z_1_dot)+S(nu)'*R'*Eta_tdot + R'*Eta_tdotdot;

    % TAU
        switch adaptation
            case 1
                tau=M_c*Alpha_1dot-diag([K_d(1,1)/sqrt([z_2(1) z_2(2)]*[z_2(1) z_2(2)]'+delta(3)^2) K_d(2,2)/sqrt([z_2(1) z_2(2)]*[z_2(1) z_2(2)]'+delta(3)^2) K_d(3,3)/sqrt(z_2(3)^2+delta(4)^2)])*z_2-theta_hat;
                theta_hat_dot = Gamma_theta*z_2;
                tau_nom=M_c*Alpha_1dot-diag([K_d(1,1)/sqrt([z_2(1) z_2(2)]*[z_2(1) z_2(2)]'+delta(3)^2) K_d(2,2)/sqrt([z_2(1) z_2(2)]*[z_2(1) z_2(2)]'+delta(3)^2) K_d(3,3)/sqrt(z_2(3)^2+delta(4)^2)])*z_2;
            otherwise
                tau=M_c*Alpha_1dot +C*Alpha_1 + D*Alpha_1 -diag([K_d(1,1)/sqrt([z_2(1) z_2(2)]*[z_2(1) z_2(2)]'+delta(3)^2) K_d(2,2)/sqrt([z_2(1) z_2(2)]*[z_2(1) z_2(2)]'+delta(3)^2) K_d(3,3)/sqrt(z_2(3)^2+delta(4)^2)])*z_2;
                theta_hat_dot = [0 0 0]';
                tau_nom=M_c*Alpha_1dot-diag([K_d(1,1)/sqrt([z_2(1) z_2(2)]*[z_2(1) z_2(2)]'+delta(3)^2) K_d(2,2)/sqrt([z_2(1) z_2(2)]*[z_2(1) z_2(2)]'+delta(3)^2) K_d(3,3)/sqrt(z_2(3)^2+delta(4)^2)])*z_2;
        end
    
         %   tau=M_c*Alpha_1dot-diag([K_d(1,1)/sqrt([z_2(1) z_2(2)]*[z_2(1) z_2(2)]'+delta(3)^2) K_d(2,2)/sqrt([z_2(1) z_2(2)]*[z_2(1) z_2(2)]'+delta(3)^2) K_d(3,3)/sqrt(z_2(3)^2+delta(4)^2)])*z_2-theta_hat;
         %   theta_hat_dot = Gamma_theta*z_2;
    case 4
        %L1 - NPNV
        
            z1=R'*(Eta_tilde);
            delta_psi = delta(1);
            delta_p = delta(2);
            delta_v = delta(3);
            delta_r = delta(4);

            z1_p = [z1(1), z1(2)]';
            z1_psi = z1(3);

            first = 1/(sqrt(z1_p'*z1_p + delta_p^2));
            second = 1/(sqrt(z1_psi^2 + delta_psi^2));

            K1 = K_p*[first*eye(2,2) zeros(2,1); zeros(1,2) second];

            Nu_d = R_T * Eta_tdot - K1 * z1;
            Alpha_1 = Nu_d;
            z2 = nu - Alpha_1;
            z2_v = [z2(1), z2(2)]';
            z2_r = z2(3);

            first2 = 1/(sqrt(z2_v'*z2_v + delta_v^2));
            second2 = 1/(sqrt(z2_r^2 + delta_r^2));

            K2 = K_d*[first2*eye(2,2) zeros(2,1); zeros(1,2) second2];
            eta_tilde = eta_hat - Eta;
            nu_tilde = nu_hat - nu;

            z1dot = S' * z1 - K1 * z1 + z2;

            z1_p = [z1(1), z1(2)]';
            z1_psi = z1(3);
            z1_pdot = [z1dot(1), z1dot(2)]';
            z1_psidot = z1dot(3);
            gamma_w_delta = (20*pi)^2/4;
            L1 = eye(3)*(2*pi)^2;%*2*K1;
            L2 = eye(3)*2*1.2*2*pi;%100;%*2*K2;

            first3 = (z1_p'*z1_pdot)/((z1_p'*z1_p + delta_p^2)^(3/2));

            second3 = (z1_psi*z1_psidot)/((z1_psi^2 + delta_psi^2)^(3/2));

            K1dot = - K_p*[first3*eye(2,2) zeros(2,1); zeros(1,2) second3];

            Alphadot = R_T * Eta_tdotdot + S_T * R_T * Eta_tdot - K1dot * z1 - K1*z1dot;
            eta_hat_dot = -L1*eta_tilde + R_T'*nu;
            nu_hat_dot = -L2*nu_tilde + M_c\(tau+w_delta_hat-C*nu-D*nu);
            tau=M_c*Alphadot+ C*Alpha_1+ D * Alpha_1 - K2 * z2 -w_delta_hat;
            w_delta_hat_dot=-gamma_w_delta*nu_tilde;
            theta_hat_dot = [0 0 0]';
            tau_nom =[0 0 0]';



        
        
%         switch adaptation
%             case 1
%                 tau=M_c*Alphadot+ D * Alpha_1 - K2 * z2 -w_delta_hat;
%                 w_delta_hat_dot=-gamma_w_delta*nu_tilde;
%                 theta_hat_dot = [0 0 0]';
%                 tau_nom =[0 0 0]';
%             otherwise
%                 tau=M_c*Alphadot+ D * Alpha_1 - K2 * z2;
%                 w_delta_hat_dot = [0 0 0]';
%                 theta_hat_dot = [0 0 0]';
%                 tau_nom =[0 0 0]';
%         end     
     case 5
        K1 = diag([0.06 0.06 0.0698]);
        K2 = diag( [0.2 0.2 0.174]*M)*4;%diag([5, 7, 15]);

        Gamma= diag([8, 4, 8, 8, 8, 4, 8, 8,0.4,0.4,0.4]);
        r = nu(3);
        v=nu(2);
        z_1 = R'*(Eta-Eta_t);


        Alpha_1 = R'*Eta_tdot - K1*z_1;

        z_2 = nu - Alpha_1;
        z_1_dot = S' * z_1 - K1 * z_1 + z_2;
        alpha_dot = R'*Eta_t_dotdot + S'*R'*Eta_tdot - K1*z_1_dot;

        Phi = [0 0 0 0 0 0 0 0; abs(r)*v r abs(v)*r abs(r)*r 0 0 0 0; 0 0 0 0 abs(r)*v r abs(v)*r abs(r)*r];
        Phi = [Phi R_T];
        phi_dot_hat = -Gamma* Phi' * ( tau- C*nu - D*nu  +  Phi*(phi_hat + Gamma*Phi'*z_2)- M_c*alpha_dot);
        %- z_1
        tau = -K2*z_2   + C*nu - D* nu  +  Phi*(phi_hat + Gamma*Phi'*z_2)- M_c*alpha_dot;          
         
    otherwise
        tau = [0 0 0]';
        tau_nom = [0 0 0]';
        z_1 = [0 0 0]';
        z_2 = [0 0 0]';
         theta_hat_dot = [0 0 0]';
         Alpha_1= [0 0 0]';
end
        
%}
tau1=tau;



%%
tau_L=[0 0 0]';
tau_U=[0 0 0]';

end

    function matrix=C_c(V) %%Coreolis matrix
    %#codegen
        matrix=C_RB_c(V)+C_A_c(V);
    end
      function matrix=C_RB_c(V)
      %#codegen
 m    = 127.92;%14.79;
 x_g  = 0;%0.0375;
 I_z  =  61.967;%1.7600;  
            u=V(1);
            v=V(2);
            r=V(3);
            matrix=[0        0       -m*(x_g*r+v);
                    0        0        m*u;
                    m*(x_g*r+v) -m*u    0]; 
      end
      function matrix=C_A_c(V)
      %#codegen
 X_ud  =    3.262; %-2.0;											% Table B.1
 Y_vd =     28.89;%-10.0;
 N_vd =    0.157;%-0.0;		% Table B.1
 Y_rd =    0.525;%  -0.0;
 N_rd =    13.98;%-1.0;		% Table B.1

            u=V(1);
            v=V(2);
            r=V(3);
        matrix=[0                                      0              Y_vd*v+0.5*(N_vd+Y_rd)*r;
               0                                       0             -X_ud*u;
               -Y_vd*v-0.5*(N_vd+Y_rd)*r         X_ud*u       0]; 
      end   
%{      
function [ d ] = G_d(nu)
      %#codegen
X_u		= -0.6555;
Y_v		= -1.33;
N_v		= 0;

    v=[nu(1) nu(2) 0]';

      D_L_uv=[-X_u    0  0 ;
            0     -Y_v 0;
            0     -N_v 0];
      d=(D_L_uv+D_NL_uv(v))*v;

end

function matrix = D_NL_uv(V)
      %#codegen


 
	
X_uu 	= 0.3545;		X_vv	= -2.443;
X_uuu 	= -3.787;	

			
Y_vv	= -2.776;			
Y_vvv	= -64.91;

N_vv	= -0.2088;	

    u=V(1);
    v=V(2);
    
     matrix=[-X_uu*abs(u)-X_uuu*u^2 0 0;
            0 -Y_vv*abs(v)-Y_vvv*v^2 0;
            0 -N_vv*abs(v) 0];
end
%}
function matrix=Rot(N)
      %#codegen

    yaw=N(3);
    matrix=[cos(yaw) -sin(yaw) 0;
            sin(yaw)  cos(yaw) 0;
            0         0        1]; 
end
%{
function R_d = Rot_dot(nu,eta)
%% takes in the nu vector 
      %#codegen


R_d=S([0 0 nu(3)])*Rot([0 0 eta(3)]);

end
%}
function [ s ] = S(r)
%UNTITLED2 Summary of this function goes here
%   Detailed explanation goes here
      %#codegen

s=[0 -r(3) r(2);
   r(3) 0 -r(1);
   -r(2) r(1) 0];

end
%{
function [ phi ] = Phi( nu )
%UNTITLED3 Summary of this function goes here
%   Detailed explanation goes here
      %#codegen

v=nu(2);
IvI=abs(v);
r=nu(3);
IrI=abs(r);

phi=[0 0 0 0 0 0 0 0;
     -IrI*v -r -IvI*r -IrI*r 0 0 0 0;
     0 0 0 0 -IrI*v -r -IvI*r -IrI*r];

end
%}

== matlab function ctrl_custom_4corner_automatic/10HZ8/MATLAB Function ==
  data: nu input; nu_10 output; nu_current input; i input; i_out output
function [nu_10,i_out] = hz(nu,nu_current,i)

if i==0
    nu_10=nu;
    i_out=1;
elseif i==10
    nu_10=nu;
    i_out=1;
else
    nu_10=nu_current;
    i_out=i+1;
end

== matlab function ctrl_custom_4corner_automatic/Complete MPAC1/MPAC Vel/MATLAB Function1 ==
  data: nu output; eta input; Phi_p input
function nu  = nu_vel(eta,Phi_p)

psi = eta(3);

R = [cos(psi) -sin(psi) 0;...
    sin(psi) cos(psi) 0;...
    0 0 1];


nu = R'*Phi_p;

== matlab function ctrl_custom_4corner_automatic/Complete MPAC1/MPAC/10HZ/MATLAB Function ==
  data: nu input; nu_10 output; nu_current input; i input; i_out output
function [nu_10,i_out] = hz(nu,nu_current,i)

if i==0
    nu_10=nu;
    i_out=1;
elseif i==10
    nu_10=nu;
    i_out=1;
else
    nu_10=nu_current;
    i_out=i+1;
end

== matlab function ctrl_custom_4corner_automatic/Complete MPAC1/MPAC/Subsystem/10HZ/MATLAB Function ==
  data: nu input; nu_10 output; nu_current input; i input; i_out output
function [nu_10,i_out] = hz(nu,nu_current,i)

if i==0
    nu_10=nu;
    i_out=1;
elseif i==10
    nu_10=nu;
    i_out=1;
else
    nu_10=nu_current;
    i_out=i+1;
end

== matlab function ctrl_custom_4corner_automatic/Saturation/MATLAB Function ==
  data: tau_c input; tau output; tau_MRS_num input; tau_MRS_block input; tau_mag input; tau_LP input; select_saturation input
function tau = fcn(tau_c,tau_MRS_num,tau_MRS_block,tau_mag,tau_LP,select_saturation)

switch select_saturation
    
    case 1
        tau = tau_c;
    case 2
        tau = tau_mag;
    case 3 
       tau = tau_MRS_block;
    case 4
        tau = tau_MRS_num;
    case 5
        tau = tau_LP;
    otherwise
        tau = [0 0 0]';
end

== matlab function ctrl_custom_4corner_automatic/Saturation1/MATLAB Function ==
  data: tau_c input; tau output; tau_MRS_num input; tau_MRS_block input; tau_mag input; tau_LP input; select_saturation input
function tau = fcn(tau_c,tau_MRS_num,tau_MRS_block,tau_mag,tau_LP,select_saturation)

switch select_saturation
    
    case 1
        tau = tau_c;
    case 2
        tau = tau_mag;
    case 3 
       tau = tau_MRS_block;
    case 4
        tau = tau_MRS_num;
    case 5
        tau = tau_LP;
    otherwise
        tau = [0 0 0]';
end

== matlab function ctrl_custom_4corner_automatic/Control/10HZ3/MATLAB Function ==
  data: nu input; nu_10 output; nu_current input; i input; i_out output
function [nu_10,i_out] = hz(nu,nu_current,i)

if i==0
    nu_10=nu;
    i_out=1;
elseif i==10
    nu_10=nu;
    i_out=1;
else
    nu_10=nu_current;
    i_out=i+1;
end

== matlab function ctrl_custom_4corner_automatic/Saturation1/MRS 1/Magnitude Constraints2 ==
  data: delta input; Tau_mrs output
function Tau_mrs = MagConstr(delta)

% mag_constr = [1.1089, 0.6387, 0.6176]; %real
mag_constr = [2, 1.5, 1]; %for lab (same ratio, but lower)

Tau_mrs = [0;0;0];

for n = 1:length(delta)
    
    if delta(n) <= -mag_constr(n)
        Tau_mrs(n) = -mag_constr(n);
    end
    
    if ((delta(n) > -mag_constr(n)) && (delta(n) < mag_constr(n)))
        Tau_mrs(n) = delta(n);
    end
    
    if delta(n) >= mag_constr(n)
        Tau_mrs(n) = mag_constr(n);
    end
    
end
    
end

== matlab function ctrl_custom_4corner_automatic/Saturation1/MRS 1/Rate Constraints1 ==
  data: epsilon input; delta_dot output
function delta_dot = RateConstr(epsilon)

rate_constr = [1.85;1.06;0.77]; %N

%By design we want to use [0.6 0.6 0.8]s from 0-->max thrust
%Based on real magnitude constraints [1.1089 0.6387 0.6176]

delta_dot = [0;0;0];

for n = 1:length(epsilon)
    
    if epsilon(n) <= -rate_constr(n)
        delta_dot(n) = -rate_constr(n);
    end
    
    if ((epsilon(n) > -rate_constr(n)) && (epsilon(n) < rate_constr(n)))
        delta_dot(n) = epsilon(n);
    end
    
    if epsilon(n) >= rate_constr(n)
        delta_dot(n) = rate_constr(n);
    end
    
end
    
end

== matlab function ctrl_custom_4corner_automatic/Saturation1/MRS_num/Magnitude Constraints2 ==
  data: delta input; Tau_mrs output
function Tau_mrs = MagConstr(delta)

% mag_constr = [1.1089, 0.6387, 0.6176]; %real
mag_constr = [1, 0.58, 0.56]; %for lab (same ratio, but lower)

Tau_mrs = [0;0;0];

for n = 1:length(delta)
    
    if delta(n) <= -mag_constr(n)
        Tau_mrs(n) = -mag_constr(n);
    end
    
    if ((delta(n) > -mag_constr(n)) && (delta(n) < mag_constr(n)))
        Tau_mrs(n) = delta(n);
    end
    
    if delta(n) >= mag_constr(n)
        Tau_mrs(n) = mag_constr(n);
    end
    
end
    
end

== matlab function ctrl_custom_4corner_automatic/Saturation1/MRS_num/Rate Constraints1 ==
  data: epsilon input; delta_dot output
function delta_dot = RateConstr(epsilon)

rate_constr = [1.85;1.06;0.77]; %N

%By design we want to use [0.6 0.6 0.8]s from 0-->max thrust
%Based on real magnitude constraints [1.1089 0.6387 0.6176]

delta_dot = [0;0;0];

for n = 1:length(epsilon)
    
    if epsilon(n) <= -rate_constr(n)
        delta_dot(n) = -rate_constr(n);
    end
    
    if ((epsilon(n) > -rate_constr(n)) && (epsilon(n) < rate_constr(n)))
        delta_dot(n) = epsilon(n);
    end
    
    if epsilon(n) >= rate_constr(n)
        delta_dot(n) = rate_constr(n);
    end
    
end
    
end

== matlab function ctrl_custom_4corner_automatic/Saturation1/MRS_num/Rate Constraints2 ==
  data: tau_c_current input; der output; tau_c_previous input
function der = derivative(tau_c_current, tau_c_previous)

der = [0;0;0];

for i=1:3
    der(i)  = (tau_c_current(i)-tau_c_previous(i))/(0.01);
end
end

== matlab function ctrl_custom_4corner_automatic/Saturation1/Magnitude Constraints2 ==
  data: Tau_c input; Tau_s output
function Tau_s = MagConstr(Tau_c)

%mag_constr = [1.1089, 0.6387, 0.6176]; %real
 mag_constr = [2, 1.5, 1]; %for lab (same ratio, but lower)

Tau_s = [0;0;0];

for n = 1:length(Tau_c)
    
    if Tau_c(n) <= -mag_constr(n)
        Tau_s(n) = -mag_constr(n);
    end
    
    if ((Tau_c(n) > -mag_constr(n)) && (Tau_c(n) < mag_constr(n)))
        Tau_s(n) = Tau_c(n);
    end
    
    if Tau_c(n) >= mag_constr(n)
        Tau_s(n) = mag_constr(n);
    end
    
end
    
end

== matlab function ctrl_custom_4corner_automatic/Subsystem1/fourcorner tracking/fourcorner tracking ==
  data: Eta_t output; Eta_t_dot output; Eta_t_ddot output; eta input; corner_switch input
function [ Eta_t, Eta_t_dot, Eta_t_ddot]   =  fourcorner_tracking(eta,corner_switch)

v_t = 0.15;

etaP = [5 7 7 7 5 5;
       -1 -1 1 1 1 -1;
        0 0 0 pi/4 pi/4 0];
Eta_t_dot = [0;0;0];
Eta_t_ddot = [0;0;0];

Eta_t = [5;-1;0];

x_threshold = 0.005;
y_threshold = 0.005;
yaw_threshold = 0.5;

persistent point ;
if(isempty(point))
    point = 1;
    
end

if(corner_switch==1)
    point =1;
end


switch point
    case 1
        Eta_t = etaP(:,2);
         if ((abs((Eta_t(1)- eta(1))) <x_threshold ) ==1  ) && ((abs(Eta_t(2)-eta(2))<y_threshold) ==1) && (abs(Eta_t(3)-rad2deg(eta(3)))<0.5 == 1)
            point = 2;
            return;
         end
        
        
    case 2
        Eta_t = etaP(:,3);
        if((abs((Eta_t(1)- eta(1))) <x_threshold ) ==1  ) && ((abs(Eta_t(2)-eta(2))<y_threshold) ==1) && (abs(Eta_t(3)-rad2deg(eta(3)))<0.5 == 1) 
            point = 3;
            return;
         end
    case 3
        Eta_t = etaP(:,4);
        if((abs((Eta_t(1)- eta(1))) <x_threshold ) ==1  ) && ((abs(Eta_t(2)-eta(2))<y_threshold) ==1) && (rad2deg(abs(Eta_t(3)-eta(3)))<0.5 == 1)  
            point = 4;
            return;
            
         end
    case 4
        Eta_t = etaP(:,5);
        if((abs((Eta_t(1)- eta(1))) <x_threshold ) ==1  ) && ((abs(Eta_t(2)-eta(2))<y_threshold) ==1) && (rad2deg(abs(Eta_t(3)-eta(3)))<0.5 == 1) 
            point = 5; 
            return;
         end
    case 5
        Eta_t = etaP(:,6);
        if((abs((Eta_t(1)- eta(1))) <x_threshold ) ==1  ) && ((abs(Eta_t(2)-eta(2))<y_threshold) ==1) && (abs(Eta_t(3)-rad2deg(eta(3)))<0.5 == 1) 
            point = 6; 
            return;
         end

    otherwise
        

end
end
%(abs(Eta_t(2)-eta(2))<0.01) &&

== matlab function ctrl_custom_4corner_automatic/Saturation/Magnitude Constraints2 ==
  data: Tau_c input; Tau_s output
function Tau_s = MagConstr(Tau_c)

%mag_constr = [1.1089, 0.6387, 0.6176]; %real
 mag_constr = [2, 1.5, 1]; %for lab (same ratio, but lower)

Tau_s = [0;0;0];

for n = 1:length(Tau_c)
    
    if Tau_c(n) <= -mag_constr(n)
        Tau_s(n) = -mag_constr(n);
    end
    
    if ((Tau_c(n) > -mag_constr(n)) && (Tau_c(n) < mag_constr(n)))
        Tau_s(n) = Tau_c(n);
    end
    
    if Tau_c(n) >= mag_constr(n)
        Tau_s(n) = mag_constr(n);
    end
    
end
    
end

== matlab function ctrl_custom_4corner_automatic/Saturation/MRS 1/Magnitude Constraints2 ==
  data: delta input; Tau_mrs output
function Tau_mrs = MagConstr(delta)

% mag_constr = [1.1089, 0.6387, 0.6176]; %real
mag_constr = [1, 0.58, 0.56]; %for lab (same ratio, but lower)

Tau_mrs = [0;0;0];

for n = 1:length(delta)
    
    if delta(n) <= -mag_constr(n)
        Tau_mrs(n) = -mag_constr(n);
    end
    
    if ((delta(n) > -mag_constr(n)) && (delta(n) < mag_constr(n)))
        Tau_mrs(n) = delta(n);
    end
    
    if delta(n) >= mag_constr(n)
        Tau_mrs(n) = mag_constr(n);
    end
    
end
    
end

== matlab function ctrl_custom_4corner_automatic/Saturation/MRS 1/Rate Constraints1 ==
  data: epsilon input; delta_dot output
function delta_dot = RateConstr(epsilon)

rate_constr = [1.85;1.06;0.77]; %N

%By design we want to use [0.6 0.6 0.8]s from 0-->max thrust
%Based on real magnitude constraints [1.1089 0.6387 0.6176]

delta_dot = [0;0;0];

for n = 1:length(epsilon)
    
    if epsilon(n) <= -rate_constr(n)
        delta_dot(n) = -rate_constr(n);
    end
    
    if ((epsilon(n) > -rate_constr(n)) && (epsilon(n) < rate_constr(n)))
        delta_dot(n) = epsilon(n);
    end
    
    if epsilon(n) >= rate_constr(n)
        delta_dot(n) = rate_constr(n);
    end
    
end
    
end

== matlab function ctrl_custom_4corner_automatic/Saturation/MRS_num/Magnitude Constraints2 ==
  data: delta input; Tau_mrs output
function Tau_mrs = MagConstr(delta)

% mag_constr = [1.1089, 0.6387, 0.6176]; %real
mag_constr = [1, 0.58, 0.56]; %for lab (same ratio, but lower)

Tau_mrs = [0;0;0];

for n = 1:length(delta)
    
    if delta(n) <= -mag_constr(n)
        Tau_mrs(n) = -mag_constr(n);
    end
    
    if ((delta(n) > -mag_constr(n)) && (delta(n) < mag_constr(n)))
        Tau_mrs(n) = delta(n);
    end
    
    if delta(n) >= mag_constr(n)
        Tau_mrs(n) = mag_constr(n);
    end
    
end
    
end

== matlab function ctrl_custom_4corner_automatic/Saturation/MRS_num/Rate Constraints1 ==
  data: epsilon input; delta_dot output
function delta_dot = RateConstr(epsilon)

rate_constr = [1.85;1.06;0.77]; %N

%By design we want to use [0.6 0.6 0.8]s from 0-->max thrust
%Based on real magnitude constraints [1.1089 0.6387 0.6176]

delta_dot = [0;0;0];

for n = 1:length(epsilon)
    
    if epsilon(n) <= -rate_constr(n)
        delta_dot(n) = -rate_constr(n);
    end
    
    if ((epsilon(n) > -rate_constr(n)) && (epsilon(n) < rate_constr(n)))
        delta_dot(n) = epsilon(n);
    end
    
    if epsilon(n) >= rate_constr(n)
        delta_dot(n) = rate_constr(n);
    end
    
end
    
end

== matlab function ctrl_custom_4corner_automatic/Saturation/MRS_num/Rate Constraints2 ==
  data: tau_c_current input; der output; tau_c_previous input
function der = derivative(tau_c_current, tau_c_previous)

der = [0;0;0];

for i=1:3
    der(i)  = (tau_c_current(i)-tau_c_previous(i))/(0.01);
end
end
